simulink model "Simulink_threshold"  (R2015a)
settings: Solver=ode45  StartTime=0.0  StopTime=10.0  RelTol=1e-3
undefined symbols (not defined in the file): gray, jet, strel
libraries: visionmorphops x2, visionsinks x2, dspvision x1
settings Model: Creator=Andrew H  LastModifiedBy=Andrew

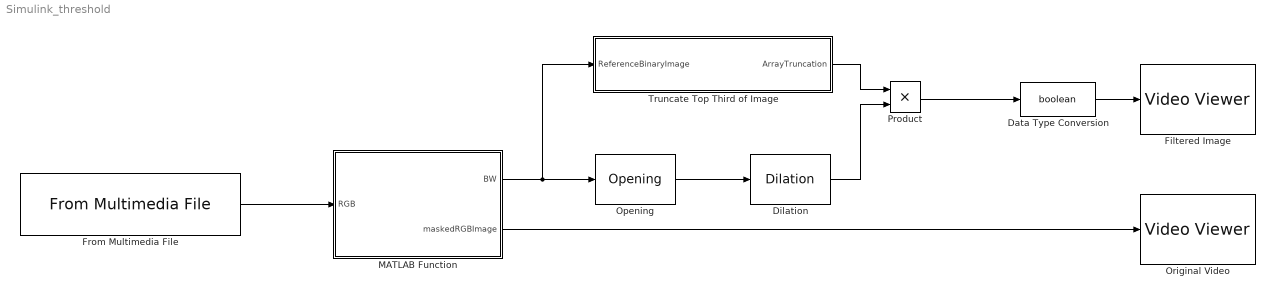
== system Simulink_threshold ==
  Data Type Conversion : DataTypeConversion  OutDataTypeStr=boolean
  Dilation : visionmorphops/Dilation  nhoodsrc=Specify via dialog  strel=[1 1; 1 1]
  Filtered Image : visionsinks/Video Viewer  inputType=Obsolete7b  imagePorts=One multidimensional signal  useColorMap=off  colormapValue=gray(256)  specRange=off  minInputVal=0  maxInputVal=255  FigPos=[962 1037 958 929]  AxisZoom=on  trueSizedOnce=off  OpenAtMdlStart=on  DefaultConfigurationName=vipscopes.VideoViewerScopeCfg
  From Multimedia File : dspvision/From Multimedia File  inputFilename=F:\Dropbox\M Eng\ECE 771 Algorithms for Paramater and State Estimation\ADAS Lane Sway Detection\rawActivity3Video.mp4  loop=on  numPlays=inf  outputStreams=Video only  videoDataType=single  audioDataType=int16  inheritSampleTime=on  userDefinedSampleTime=1/30  noAudioOutput=off  isIntensityVideo=off  fourcc=RGB  colorVideoFormat=One multidimensional signal  outputEOF=off  dataOrg=Column-major  audioFrameSize=1024  computeAudioFrameSize=off  outSamplingMode=Sample based
  MATLAB Function : MATLAB Function  TreatAsAtomicUnit=on
  Opening : visionmorphops/Opening  nhoodsrc=Specify via dialog  strel=strel('disk', 1)
  Original Video : visionsinks/Video Viewer  inputType=Obsolete7b  imagePorts=One multidimensional signal  useColorMap=off  colormapValue=jet(256)  specRange=off  minInputVal=0  maxInputVal=255  FigPos=[2 1037 958 929]  AxisZoom=on  trueSizedOnce=off  OpenAtMdlStart=on  DefaultConfigurationName=vipscopes.VideoViewerScopeCfg
  Product : Product
  Truncate Top Third of Image : MATLAB Function  TreatAsAtomicUnit=on
  wires:
  From Multimedia File/1 -> MATLAB Function/1(RGB)
  MATLAB Function/1(BW) -> Truncate Top Third of Image/1(ReferenceBinaryImage), Opening/1
  Opening/1 -> Dilation/1
  MATLAB Function/2(maskedRGBImage) -> Original Video/1
  Truncate Top Third of Image/1(ArrayTruncation) -> Product/1
  Dilation/1 -> Product/2
  Product/1 -> Data Type Conversion/1
  Data Type Conversion/1 -> Filtered Image/1

== matlab function Simulink_threshold/Truncate Top Third of Image ==
  data: ReferenceBinaryImage input; ArrayTruncation output
function ArrayTruncation = fcn(ReferenceBinaryImage)

%This function truncates the image you are processing by O variable fraction.
% In this case, O was set to 3 and deletes the first third of the flattened
% 2D array.

O = 3/10; %1/3 1/2 4/10

[x,y] = size(ReferenceBinaryImage);
matrix = zeros(x, y);

for i = x*O:x
    for j = 1:y
        matrix(i,j) = 1;
    end
end

ArrayTruncation = matrix;

end

== matlab function Simulink_threshold/MATLAB Function ==
  data: RGB input; BW output; maskedRGBImage output
function [BW,maskedRGBImage] = createMask(RGB)

% Outputs a BW (binary image) and maskedRGBImage (threshold set using the
% colorThresholder app) from a image/video frame.

%createMask  Threshold RGB image using auto-generated code from colorThresholder app.
%  [BW,MASKEDRGBIMAGE] = createMask(RGB) thresholds image RGB using
%  auto-generated code from the colorThresholder App. The colorspace and
%  minimum/maximum values for each channel of the colorspace were set in the
%  App and result in a binary mask BW and a composite image maskedRGBImage,
%  which shows the original RGB image values under the mask BW.

% Auto-generated by colorThresholder app on 14-Oct-2015
%------------------------------------------------------

% Convert RGB image to chosen color space
I = rgb2hsv(RGB);

% Define thresholds for channel 1 based on histogram settings
channel1Min = 0.952;
channel1Max = 0.094;

% Define thresholds for channel 2 based on histogram settings
channel2Min = 0.025;
channel2Max = 1.000;

% Define thresholds for channel 3 based on histogram settings
channel3Min = 0.724;
channel3Max = 0.967;

% Create mask based on chosen histogram thresholds
BW = ( (I(:,:,1) >= channel1Min) | (I(:,:,1) <= channel1Max) ) & ...
    (I(:,:,2) >= channel2Min ) & (I(:,:,2) <= channel2Max) & ...
    (I(:,:,3) >= channel3Min ) & (I(:,:,3) <= channel3Max);

% Initialize output masked image based on input image.
maskedRGBImage = RGB;

% Set background pixels where BW is false to zero.
maskedRGBImage(repmat(~BW,[1 1 3])) = 0;



% My original Code threshold block
% % Convert RGB image to chosen color space
% I = rgb2hsv(RGB);
% 
% % Define thresholds for channel 1 based on histogram settings
% channel1Min = 0.982;
% channel1Max = 0.235;
% 
% % Define thresholds for channel 2 based on histogram settings
% channel2Min = 0.043;
% channel2Max = 0.655;
% 
% % Define thresholds for channel 3 based on histogram settings
% channel3Min = 0.600;
% channel3Max = 1.000;
% 
% % Create mask based on chosen histogram thresholds
% BW = ( (I(:,:,1) >= channel1Min) | (I(:,:,1) <= channel1Max) ) & ...
%     (I(:,:,2) >= channel2Min ) & (I(:,:,2) <= channel2Max) & ...
%     (I(:,:,3) >= channel3Min ) & (I(:,:,3) <= channel3Max);
% 
% % Initialize output masked image based on input image.
% maskedRGBImage = RGB;
% 
% % Set background pixels where BW is false to zero.
% maskedRGBImage(repmat(~BW,[1 1 3])) = 0;
